simulink model "planta4tanques"  (R2013b)
settings: Solver=ode45  StartTime=0.0  StopTime=50  RelTol=1e-3
values from neighbouring files (symbols this model uses):
  A_ = 47.6    [planta4tanquesParametros.m]
  g = 978    [planta4tanquesParametros.m]
undefined symbols (not defined in the file or in its folder): A, a1, a2, a3, a4, B, C, D, gamma1, gamma2, h1_, h2_, h3_, h4_, k1, k2, step_time_1, step_time_2, v1_, v1_f, v1_i, v2_, v2_f, v2_i
settings Model: Creator=Samsung  LastModifiedBy=Samsung

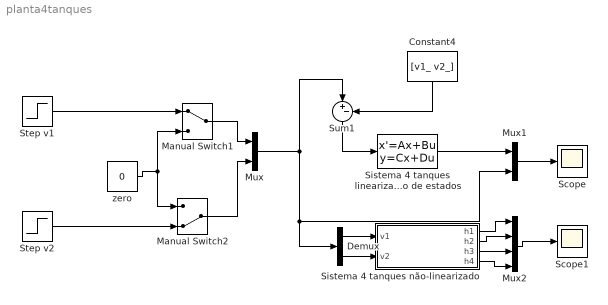
== system planta4tanques ==
  Constant4 : Constant  Value=[v1_ v2_]
  Demux : Demux  Outputs=2
  Manual Switch1 : ManualSwitch
  Manual Switch2 : ManualSwitch  CurrentSetting=0
  Mux : Mux  Inputs=2
  Mux1 : Mux  Inputs=2
  Mux2 : Mux
  Scope : Scope
  Scope1 : Scope
      settings: SaveName=ScopeData9
  Sistema 4 tanques linearizado Espaço de estados : StateSpace  A=A  B=B  C=C  D=D  X0=[h1_ h2_ h3_ h4_]
  Sistema 4 tanques não-linearizado : Subsystem
  "Step v2 " : Step  Time=step_time_2  Before=v2_i  After=v2_f  SampleTime=0
  Step v1 : Step  Time=step_time_1  Before=v1_i  After=v1_f  SampleTime=0
  Sum1 : Sum  Inputs=|+-  SaturateOnIntegerOverflow=on
  "zero " : Constant  Value=0
  wires:
  Mux1/1 -> Scope/1
  Demux/2 -> Sistema 4 tanques não-linearizado/2(v2)
  Demux/1 -> Sistema 4 tanques não-linearizado/1("v1 ")
  Mux2/1 -> Scope1/1
  "zero "/1 -> Manual Switch1/2, Manual Switch2/1
  "Step v2 "/1 -> Manual Switch2/2
  Manual Switch1/1 -> Mux/1
  Manual Switch2/1 -> Mux/2
  Sistema 4 tanques não-linearizado/1(h1) -> Mux2/1
  Sistema 4 tanques não-linearizado/2(h2) -> Mux2/2
  Sistema 4 tanques não-linearizado/3(h3) -> Mux2/3
  Sistema 4 tanques não-linearizado/4(h4) -> Mux2/4
  Sistema 4 tanques linearizado Espaço de estados/1 -> Mux1/1
  Step v1/1 -> Manual Switch1/1
  Constant4/1 -> Sum1/2
  Mux/1 -> Sum1/1, Mux1/2, Demux/1
  Sum1/1 -> Sistema 4 tanques linearizado Espaço de estados/1

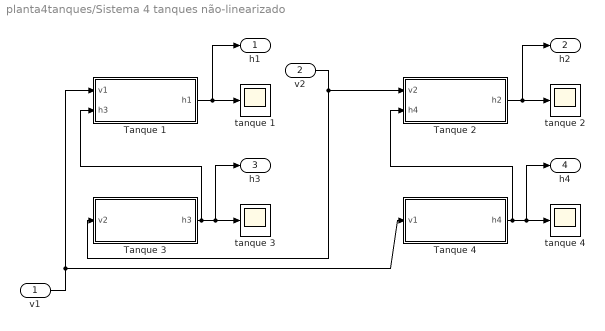
== system planta4tanques/Sistema 4 tanques não-linearizado ==
  "v1 " : Inport
  v2 : Inport  Port=2
  Tanque 1 : Subsystem
  Tanque 2 : Subsystem
  Tanque 3 : Subsystem
  Tanque 4 : Subsystem
  tanque {1..4} (4 alike) : Scope
      tanque 1 settings: TimeRange=500  YMin=0  YMax=0.16  SaveName=ScopeData5
      tanque 2 settings: TimeRange=500  YMin=0  YMax=0.16  SaveName=ScopeData6
      tanque 3 settings: TimeRange=500  YMin=0  YMax=0.16  SaveName=ScopeData7
      tanque 4 settings: TimeRange=500  YMin=0  YMax=0.16  SaveName=ScopeData8
  h1 : Outport
  h2 : Outport  Port=2
  h3 : Outport  Port=3
  h4 : Outport  Port=4
  wires:
  Tanque 3/1("h3 ") -> h3/1, tanque 3/1, Tanque 1/2(h3)
  Tanque 4/1(h4) -> h4/1, tanque 4/1, Tanque 2/2(h4)
  "v1 "/1 -> Tanque 1/1("v1 "), Tanque 4/1(v1)
  v2/1 -> Tanque 3/1(v2), Tanque 2/1(v2)
  Tanque 1/1(h1) -> h1/1, tanque 1/1
  Tanque 2/1(h2) -> h2/1, tanque 2/1

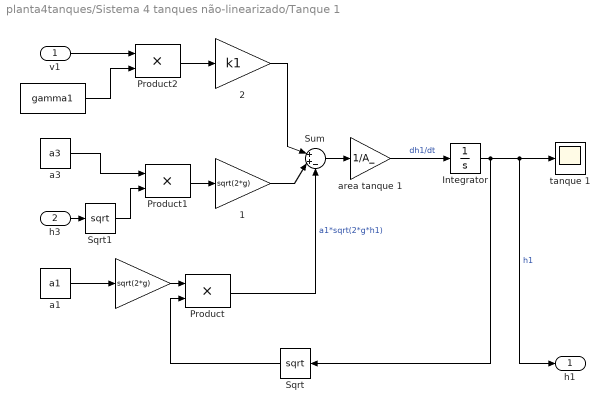
== system planta4tanques/Sistema 4 tanques não-linearizado/Tanque 1 ==
  "v1 " : Inport
  h3 : Inport  Port=2
  " " : Constant  Value=gamma1
  " " : Gain  Gain=sqrt(2*g)  SaturateOnIntegerOverflow=on  OutDataTypeStr=Inherit: Same as input  ParamDataTypeStr=Inherit: Same as input
  " 1" : Gain  Gain=sqrt(2*g)  SaturateOnIntegerOverflow=on  OutDataTypeStr=Inherit: Same as input  ParamDataTypeStr=Inherit: Same as input
  " 2" : Gain  Gain=k1  SaturateOnIntegerOverflow=on  OutDataTypeStr=Inherit: Same as input  ParamDataTypeStr=Inherit: Same as input
  " a1" : Constant  Value=a1
  " a3" : Constant  Value=a3
  Integrator : Integrator  InitialCondition=h1_
  Product : Product  SaturateOnIntegerOverflow=on  OutDataTypeStr=Inherit: Same as first input
  Product1 : Product  SaturateOnIntegerOverflow=on  OutDataTypeStr=Inherit: Same as first input
  Product2 : Product  SaturateOnIntegerOverflow=on  OutDataTypeStr=Inherit: Same as first input
  Sqrt : Sqrt  SaturateOnIntegerOverflow=on
  Sqrt1 : Sqrt  SaturateOnIntegerOverflow=on
  Sum : Sum  Inputs=|++-
  area tanque 1 : Gain  Gain=1/A_
  "tanque 1 " : Scope
      settings: TimeRange=500  YMin=0  YMax=0.16
  h1 : Outport
  wires:
  Sum/1 -> area tanque 1/1
  area tanque 1/1 -> Integrator/1  "dh1/dt"
  Sqrt/1 -> Product/2
  Integrator/1 -> Sqrt/1, h1/1, "tanque 1 "/1  "h1"
  " a1"/1 -> " "/1
  " "/1 -> Product/1
  Product/1 -> Sum/3  "a1*sqrt(2*g*h1)"
  Product1/1 -> " 1"/1
  " a3"/1 -> Product1/1
  Sqrt1/1 -> Product1/2
  h3/1 -> Sqrt1/1
  " 1"/1 -> Sum/2
  " "/1 -> Product2/2
  "v1 "/1 -> Product2/1
  Product2/1 -> " 2"/1
  " 2"/1 -> Sum/1

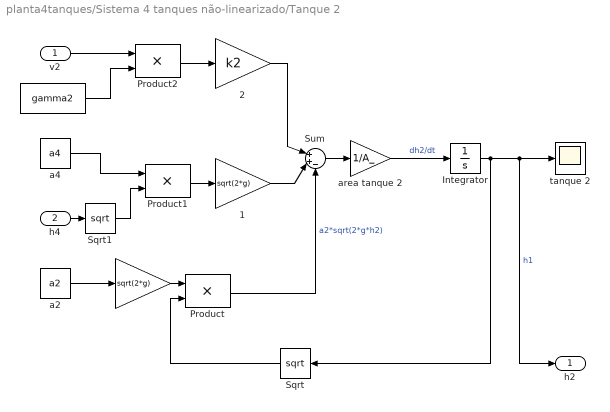
== system planta4tanques/Sistema 4 tanques não-linearizado/Tanque 2 ==
  v2 : Inport
  h4 : Inport  Port=2
  " " : Constant  Value=gamma2
  " " : Gain  Gain=sqrt(2*g)  SaturateOnIntegerOverflow=on  OutDataTypeStr=Inherit: Same as input  ParamDataTypeStr=Inherit: Same as input
  " 1" : Gain  Gain=sqrt(2*g)  SaturateOnIntegerOverflow=on  OutDataTypeStr=Inherit: Same as input  ParamDataTypeStr=Inherit: Same as input
  " 2" : Gain  Gain=k2  SaturateOnIntegerOverflow=on  OutDataTypeStr=Inherit: Same as input  ParamDataTypeStr=Inherit: Same as input
  " a2" : Constant  Value=a2
  " a4" : Constant  Value=a4
  Integrator : Integrator
  Product : Product  SaturateOnIntegerOverflow=on  OutDataTypeStr=Inherit: Same as first input
  Product1 : Product  SaturateOnIntegerOverflow=on  OutDataTypeStr=Inherit: Same as first input
  Product2 : Product  SaturateOnIntegerOverflow=on  OutDataTypeStr=Inherit: Same as first input
  Sqrt : Sqrt  SaturateOnIntegerOverflow=on
  Sqrt1 : Sqrt  SaturateOnIntegerOverflow=on
  Sum : Sum  Inputs=|++-
  area tanque 2 : Gain  Gain=1/A_
  "tanque 2 " : Scope
      settings: TimeRange=500  YMin=0  YMax=0.16  SaveName=ScopeData2
  h2 : Outport
  wires:
  Sum/1 -> area tanque 2/1
  area tanque 2/1 -> Integrator/1  "dh2/dt"
  Sqrt/1 -> Product/2
  Integrator/1 -> Sqrt/1, h2/1, "tanque 2 "/1  "h1"
  " a2"/1 -> " "/1
  " "/1 -> Product/1
  Product/1 -> Sum/3  "a2*sqrt(2*g*h2)"
  Product1/1 -> " 1"/1
  " a4"/1 -> Product1/1
  Sqrt1/1 -> Product1/2
  h4/1 -> Sqrt1/1
  " 1"/1 -> Sum/2
  " "/1 -> Product2/2
  v2/1 -> Product2/1
  Product2/1 -> " 2"/1
  " 2"/1 -> Sum/1

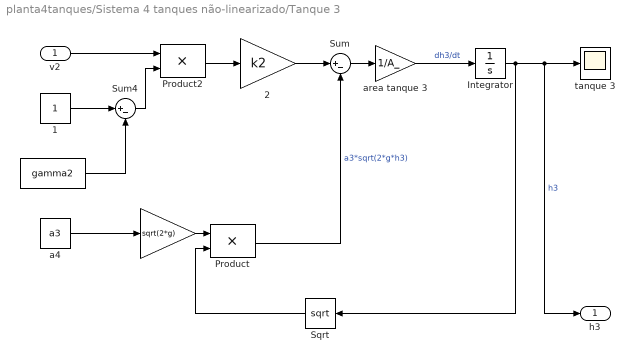
== system planta4tanques/Sistema 4 tanques não-linearizado/Tanque 3 ==
  v2 : Inport
  " " : Constant  Value=gamma2
  " " : Gain  Gain=sqrt(2*g)  SaturateOnIntegerOverflow=on  OutDataTypeStr=Inherit: Same as input  ParamDataTypeStr=Inherit: Same as input
  " 2" : Gain  Gain=k2  SaturateOnIntegerOverflow=on  OutDataTypeStr=Inherit: Same as input  ParamDataTypeStr=Inherit: Same as input
  " 1" : Constant
  " a4" : Constant  Value=a3
  Integrator : Integrator
  Product : Product  SaturateOnIntegerOverflow=on  OutDataTypeStr=Inherit: Same as first input
  Product2 : Product  SaturateOnIntegerOverflow=on  OutDataTypeStr=Inherit: Same as first input
  Sqrt : Sqrt  SaturateOnIntegerOverflow=on
  Sum : Sum  Inputs=|+-
  Sum4 : Sum  Inputs=|+-  SaturateOnIntegerOverflow=on
  area tanque 3 : Gain  Gain=1/A_
  "tanque 3 " : Scope
      settings: TimeRange=500  YMin=0  YMax=0.16  SaveName=ScopeData3
  "h3 " : Outport
  wires:
  Sum/1 -> area tanque 3/1
  area tanque 3/1 -> Integrator/1  "dh3/dt"
  Sqrt/1 -> Product/2
  Integrator/1 -> Sqrt/1, "h3 "/1, "tanque 3 "/1  "h3"
  " a4"/1 -> " "/1
  " "/1 -> Product/1
  Product/1 -> Sum/2  "a3*sqrt(2*g*h3)"
  v2/1 -> Product2/1
  Product2/1 -> " 2"/1
  " 2"/1 -> Sum/1
  " "/1 -> Sum4/2
  " 1"/1 -> Sum4/1
  Sum4/1 -> Product2/2

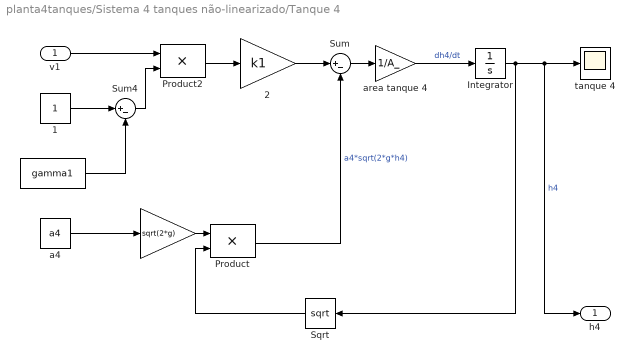
== system planta4tanques/Sistema 4 tanques não-linearizado/Tanque 4 ==
  v1 : Inport
  " " : Constant  Value=gamma1
  " " : Gain  Gain=sqrt(2*g)  SaturateOnIntegerOverflow=on  OutDataTypeStr=Inherit: Same as input  ParamDataTypeStr=Inherit: Same as input
  " 2" : Gain  Gain=k1  SaturateOnIntegerOverflow=on  OutDataTypeStr=Inherit: Same as input  ParamDataTypeStr=Inherit: Same as input
  " 1" : Constant
  " a4" : Constant  Value=a4
  Integrator : Integrator
  Product : Product  SaturateOnIntegerOverflow=on  OutDataTypeStr=Inherit: Same as first input
  Product2 : Product  SaturateOnIntegerOverflow=on  OutDataTypeStr=Inherit: Same as first input
  Sqrt : Sqrt  SaturateOnIntegerOverflow=on
  Sum : Sum  Inputs=|+-
  Sum4 : Sum  Inputs=|+-  SaturateOnIntegerOverflow=on
  area tanque 4 : Gain  Gain=1/A_
  "tanque 4 " : Scope
      settings: TimeRange=500  YMin=0  YMax=0.16  SaveName=ScopeData4
  h4 : Outport
  wires:
  Sum/1 -> area tanque 4/1
  area tanque 4/1 -> Integrator/1  "dh4/dt"
  Sqrt/1 -> Product/2
  Integrator/1 -> Sqrt/1, h4/1, "tanque 4 "/1  "h4"
  " a4"/1 -> " "/1
  " "/1 -> Product/1
  Product/1 -> Sum/2  "a4*sqrt(2*g*h4)"
  v1/1 -> Product2/1
  Product2/1 -> " 2"/1
  " 2"/1 -> Sum/1
  " "/1 -> Sum4/2
  " 1"/1 -> Sum4/1
  Sum4/1 -> Product2/2
